simulink model "test"  (R2021b)
settings: Solver=ode1  StartTime=0.0  StopTime=20.0  FixedStep=0.01  RelTol=1e-3
PreLoadFcn:
  | if exist('tl_preloadfcn','file'), tl_preloadfcn(gcs,'5.2.0.25'); end
  | 
  | sDataDefFile = ''; %Empty -> Data Generated into Model source file
  | %% Signal driver_up
  | driver_up = Simulink.Signal;
  | driver_up.DataType = 'boolean';
  | driver_up.Min = 0;
  | driver_up.Max = 1;
  | driver_up.CoderInfo.StorageClass = 'Custom';
  | driver_up.CoderInfo.CustomStorageClass = 'ExportToFile';
  | driver_up.CoderInfo.CustomAttributes.DefinitionFile = sDataDefFile;
  | %% Parameter auto_up_time
  | auto_up_time            = Simulink.Parameter;
  | auto_up_time.Value      = 100;
  | auto_up_time.DataType   = 'uint8';
  | auto_up_time.Min        = 0;
  | auto_up_time.Max        = 255;
  | auto_up_time.CoderInfo.StorageClass = 'Custom';
  | auto_up_time.CoderInfo.CustomStorageClass = 'ConstVolatile';
  | auto_up_time.CoderInfo.CustomAttributes.DefinitionFile = sDataDefFile;
  | %% Signal driver_down
  | driver_down                 = copy(driver_up);
  | %% Signal passenger_up
  | passenger_up                = copy(driver_up);
  | %% Signal passenger_down
  | passenger_down              = copy(driver_up);
  | move_up                     = copy(driver_up);
  | move_down                   = copy(driver_up);
  | obstacle_detection          = copy(driver_up);
  | driver_validated_neutral    = copy(driver_up);
  | driver_validated_up         = copy(driver_up);
  | driver_validated_down       = copy(driver_up);
  | passenger_validated_neutral = copy(driver_up);
  | passenger_validated_up      = copy(driver_up);
  | passenger_validated_down    = copy(driver_up);
  | endstop_top                 = copy(driver_up);
  | endstop_bottom              = copy(driver_up);
  | prev_move_up                = copy(driver_up);
  | obstacle_position = Simulink.Signal;
  | obstacle_position.DataType = 'fixdt(0,16,0.001,0)';
  | obstacle_position.Min = 0;
  | obstacle_position.Max = 0.45;
  | obstacle_position.CoderInfo.StorageClass        = 'Custom';
  | obstacle_position.CoderInfo.CustomStorageClass  = 'ExportToFile';
  | obstacle_position.CoderInfo.CustomAttributes.DefinitionFile = sDataDefFile;
  | 
  | window_position = copy(obstacle_position);
  | 
  | %% Parameters (Global Const Volatile)
  | position_endstop_top            = Simulink.Parameter;
  | position_endstop_top.Value      = 0.4;
  | position_endstop_top.DataType   = 'fixdt(0,16,0.001,0)';
  | position_endstop_top.Min        = 0.35;
  | position_endstop_top.Max        = 0.45;
  | position_endstop_top.CoderInfo.StorageClass = 'Custom';
  | position_endstop_top.CoderInfo.CustomStorageClass = 'ConstVolatile';
  | position_endstop_top.CoderInfo.CustomAttributes.DefinitionFile = sDataDefFile;
  | auto_down_time = copy(auto_up_time);
  | emergency_down_time = copy(auto_up_time);
  | %% Constant
  | ... (+7 lines)
PostLoadFcn:
  | if exist('tl_postloadfcn','file'), tl_postloadfcn(gcs,'5.2.0.25'); end
InitFcn:
  | if exist('tlds_init','file'), tlds_init(gcs); end
StartFcn:
  | if exist('tlds_start','file'), tlds_start(gcs); end
StopFcn:
  | if exist('tlds_stop','file'), tlds_stop(gcs); end
libraries: tllib x7
(part 2 of 2)

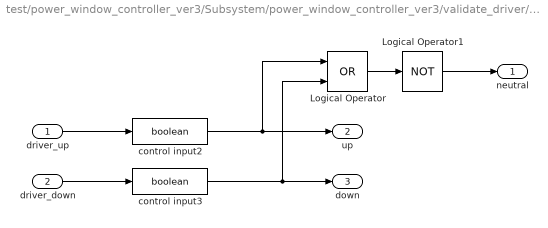
== system test/power_window_controller_ver3/Subsystem/power_window_controller_ver3/validate_driver/driver_switch ==
  driver_up : Inport  RequirementInfo={} %GIDa_88509d42_ace7_45cf_b2c2_89e39ae0ed2c
  driver_down : Inport  RequirementInfo={} %GIDa_beb14dc3_344f_4742_a2d0_fd6ea4a2bf32  Port=2
  Logical Operator : Logic  RequirementInfo={} %GIDa_da5550dd_f94c_4b73_b961_4a47a5203149  Operator=OR  AllPortsSameDT=off  OutDataTypeStr=boolean  mask(TL_LogicalOperator){data={'date',735992.62219250004}}
      settings: CopyFcn=if exist('copy_tlblock','file')==2,copy_tlblock(gcbh);end  DeleteFcn=if exist('delete_tlblock','file')==2,delete_tlblock(gcbh);end  NameChangeFcn=if exist('rename_tlblock','file')==2,rename_tlblock(gcbh);end  OpenFcn=if exist('tl_open_blockdlg','file')==2,tl_open_blockdlg(gcbh);else,open_system(gcbh,'parameter');end
      mask Help: eval(['if exist(''tl_online_help'',''file'') == 2, tl_online_help(''Topic'',''TL_LogicalOperator''),else, web([''jar:file:///'',matlabroot,''/help/toolbox/simulink/help.jar!/slref/' lower(get_param(gcbh,'Blocktype')) '.html''], ''-helpbrowser''),end'])
      mask Display:
      | [x,y] = tlDrawBrandOnBlockIcon(gcbh);
      | plot(x,y);
  Logical Operator1 : Logic  RequirementInfo={} %GIDa_999e8679_8f6d_4720_ab4a_29693e123b6b  Operator=NOT  Inputs=1  AllPortsSameDT=off  OutDataTypeStr=boolean  mask(TL_LogicalOperator){data={'date',735992.62266063655}}
      settings: CopyFcn=if exist('copy_tlblock','file')==2,copy_tlblock(gcbh);end  DeleteFcn=if exist('delete_tlblock','file')==2,delete_tlblock(gcbh);end  NameChangeFcn=if exist('rename_tlblock','file')==2,rename_tlblock(gcbh);end  OpenFcn=if exist('tl_open_blockdlg','file')==2,tl_open_blockdlg(gcbh);else,open_system(gcbh,'parameter');end
      mask Help: eval(['if exist(''tl_online_help'',''file'') == 2, tl_online_help(''Topic'',''TL_LogicalOperator''),else, web([''jar:file:///'',matlabroot,''/help/toolbox/simulink/help.jar!/slref/' lower(get_param(gcbh,'Blocktype')) '.html''], ''-helpbrowser''),end'])
      mask Display:
      | [x,y] = tlDrawBrandOnBlockIcon(gcbh);
      | plot(x,y);
  control input2 : DataTypeConversion  RequirementInfo={} %GIDa_1fd256de_8139_439f_b8bd_b0cd16c1aab9  OutDataTypeStr=boolean  SaturateOnIntegerOverflow=on  RndMeth=Zero  mask(TL_Rescaler){data={'date',730486}}
      settings: CopyFcn=if exist('copy_tlblock','file')==2,copy_tlblock(gcbh);end  DeleteFcn=if exist('delete_tlblock','file')==2,delete_tlblock(gcbh);end  NameChangeFcn=if exist('rename_tlblock','file')==2,rename_tlblock(gcbh);end  OpenFcn=if exist('tl_open_blockdlg','file')==2,tl_open_blockdlg(gcbh);else,open_system(gcbh,'parameter');end
      mask Help: eval(['if exist(''tl_online_help'',''file'') == 2, tl_online_help(''Topic'',''TL_Rescaler''),else, web([''jar:file:///'',matlabroot,''/help/toolbox/simulink/help.jar!/slref/' lower(get_param(gcbh,'Blocktype')) '.html''], ''-helpbrowser''),end'])
      mask Display:
      | [x,y] = tlDrawBrandOnBlockIcon(gcbh);
      | plot(x,y);
  control input3 : DataTypeConversion  RequirementInfo={} %GIDa_36784b95_c4a4_49da_bf15_3958bcd12f2f  OutDataTypeStr=boolean  SaturateOnIntegerOverflow=on  RndMeth=Zero  mask(TL_Rescaler){data={'date',730486}}
      settings: CopyFcn=if exist('copy_tlblock','file')==2,copy_tlblock(gcbh);end  DeleteFcn=if exist('delete_tlblock','file')==2,delete_tlblock(gcbh);end  NameChangeFcn=if exist('rename_tlblock','file')==2,rename_tlblock(gcbh);end  OpenFcn=if exist('tl_open_blockdlg','file')==2,tl_open_blockdlg(gcbh);else,open_system(gcbh,'parameter');end
      mask Help: eval(['if exist(''tl_online_help'',''file'') == 2, tl_online_help(''Topic'',''TL_Rescaler''),else, web([''jar:file:///'',matlabroot,''/help/toolbox/simulink/help.jar!/slref/' lower(get_param(gcbh,'Blocktype')) '.html''], ''-helpbrowser''),end'])
      mask Display:
      | [x,y] = tlDrawBrandOnBlockIcon(gcbh);
      | plot(x,y);
  neutral : Outport  RequirementInfo={} %GIDa_52397442_78d7_49fa_a893_524ae7078fcb  VectorParamsAs1DForOutWhenUnconnected=off
  up : Outport  RequirementInfo={} %GIDa_11ca0414_1b98_43c5_8236_d6cb17915be3  Port=2  VectorParamsAs1DForOutWhenUnconnected=off
  down : Outport  RequirementInfo={} %GIDa_c006668c_2a8f_411c_a55d_2fcf10c84114  Port=3  VectorParamsAs1DForOutWhenUnconnected=off
  wires:
  Logical Operator1/1 -> neutral/1
  Logical Operator/1 -> Logical Operator1/1
  control input3/1 -> Logical Operator/2, down/1
  control input2/1 -> Logical Operator/1, up/1
  driver_down/1 -> control input3/1
  driver_up/1 -> control input2/1

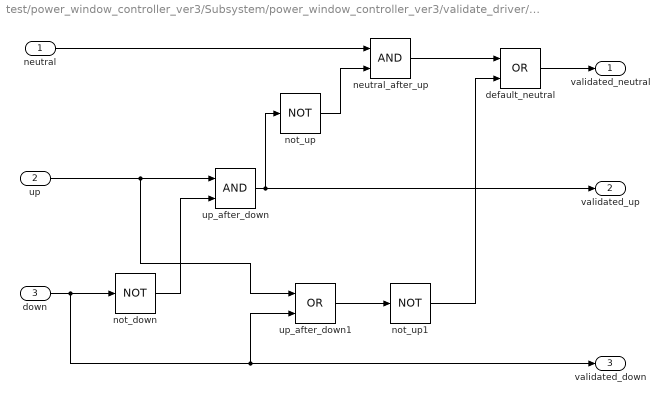
== system test/power_window_controller_ver3/Subsystem/power_window_controller_ver3/validate_driver/mutually_exclusive ==
  neutral : Inport  RequirementInfo={} %GIDa_383a4fa9_ecde_419e_b29b_a733e5593bc2
  up : Inport  RequirementInfo={} %GIDa_3190656b_05c4_4e8f_afb6_15ac29bcab83  Port=2
  down : Inport  RequirementInfo={} %GIDa_9b767e83_1086_482d_996f_d13516317d5e  Port=3
  default_neutral : Logic  RequirementInfo={} %GIDa_d3e9b556_6fe4_4d4f_868e_156175e008c8  Operator=OR  AllPortsSameDT=off  OutDataTypeStr=boolean  mask(TL_LogicalOperator){data={'date',735992.62933622685}}
      settings: CopyFcn=if exist('copy_tlblock','file')==2,copy_tlblock(gcbh);end  DeleteFcn=if exist('delete_tlblock','file')==2,delete_tlblock(gcbh);end  NameChangeFcn=if exist('rename_tlblock','file')==2,rename_tlblock(gcbh);end  OpenFcn=if exist('tl_open_blockdlg','file')==2,tl_open_blockdlg(gcbh);else,open_system(gcbh,'parameter');end
      mask Help: eval(['if exist(''tl_online_help'',''file'') == 2, tl_online_help(''Topic'',''TL_LogicalOperator''),else, web([''jar:file:///'',matlabroot,''/help/toolbox/simulink/help.jar!/slref/' lower(get_param(gcbh,'Blocktype')) '.html''], ''-helpbrowser''),end'])
      mask Display:
      | [x,y] = tlDrawBrandOnBlockIcon(gcbh);
      | plot(x,y);
  neutral_after_up : Logic  RequirementInfo={} %GIDa_2a0ebed4_26f4_4b16_ab66_395a1ddbb03e  AllPortsSameDT=off  OutDataTypeStr=boolean  mask(TL_LogicalOperator){data={'date',730486}}
      settings: CopyFcn=if exist('copy_tlblock','file')==2,copy_tlblock(gcbh);end  DeleteFcn=if exist('delete_tlblock','file')==2,delete_tlblock(gcbh);end  NameChangeFcn=if exist('rename_tlblock','file')==2,rename_tlblock(gcbh);end  OpenFcn=if exist('tl_open_blockdlg','file')==2,tl_open_blockdlg(gcbh);else,open_system(gcbh,'parameter');end
      mask Help: eval(['if exist(''tl_online_help'',''file'') == 2, tl_online_help(''Topic'',''TL_LogicalOperator''),else, web([''jar:file:///'',matlabroot,''/help/toolbox/simulink/help.jar!/slref/' lower(get_param(gcbh,'Blocktype')) '.html''], ''-helpbrowser''),end'])
      mask Display:
      | [x,y] = tlDrawBrandOnBlockIcon(gcbh);
      | plot(x,y);
  not_down : Logic  RequirementInfo={} %GIDa_717def5e_3a6b_41f3_97d3_f7d9ab03bba7  Operator=NOT  Inputs=1  AllPortsSameDT=off  OutDataTypeStr=boolean  mask(TL_LogicalOperator){data={'date',735992.6300086343}}
      settings: CopyFcn=if exist('copy_tlblock','file')==2,copy_tlblock(gcbh);end  DeleteFcn=if exist('delete_tlblock','file')==2,delete_tlblock(gcbh);end  NameChangeFcn=if exist('rename_tlblock','file')==2,rename_tlblock(gcbh);end  OpenFcn=if exist('tl_open_blockdlg','file')==2,tl_open_blockdlg(gcbh);else,open_system(gcbh,'parameter');end
      mask Help: eval(['if exist(''tl_online_help'',''file'') == 2, tl_online_help(''Topic'',''TL_LogicalOperator''),else, web([''jar:file:///'',matlabroot,''/help/toolbox/simulink/help.jar!/slref/' lower(get_param(gcbh,'Blocktype')) '.html''], ''-helpbrowser''),end'])
      mask Display:
      | [x,y] = tlDrawBrandOnBlockIcon(gcbh);
      | plot(x,y);
  not_up : Logic  RequirementInfo={} %GIDa_639c22ba_cf00_4eaa_845a_300072015885  Operator=NOT  Inputs=1  AllPortsSameDT=off  OutDataTypeStr=boolean  mask(TL_LogicalOperator){data={'date',735992.62898631941}}
      settings: CopyFcn=if exist('copy_tlblock','file')==2,copy_tlblock(gcbh);end  DeleteFcn=if exist('delete_tlblock','file')==2,delete_tlblock(gcbh);end  NameChangeFcn=if exist('rename_tlblock','file')==2,rename_tlblock(gcbh);end  OpenFcn=if exist('tl_open_blockdlg','file')==2,tl_open_blockdlg(gcbh);else,open_system(gcbh,'parameter');end
      mask Help: eval(['if exist(''tl_online_help'',''file'') == 2, tl_online_help(''Topic'',''TL_LogicalOperator''),else, web([''jar:file:///'',matlabroot,''/help/toolbox/simulink/help.jar!/slref/' lower(get_param(gcbh,'Blocktype')) '.html''], ''-helpbrowser''),end'])
      mask Display:
      | [x,y] = tlDrawBrandOnBlockIcon(gcbh);
      | plot(x,y);
  not_up1 : Logic  RequirementInfo={} %GIDa_b9044636_34db_4ac8_92ea_fff124b8872b  Operator=NOT  Inputs=1  AllPortsSameDT=off  OutDataTypeStr=boolean  mask(TL_LogicalOperator){data={'date',735992.62922876154}}
      settings: CopyFcn=if exist('copy_tlblock','file')==2,copy_tlblock(gcbh);end  DeleteFcn=if exist('delete_tlblock','file')==2,delete_tlblock(gcbh);end  NameChangeFcn=if exist('rename_tlblock','file')==2,rename_tlblock(gcbh);end  OpenFcn=if exist('tl_open_blockdlg','file')==2,tl_open_blockdlg(gcbh);else,open_system(gcbh,'parameter');end
      mask Help: eval(['if exist(''tl_online_help'',''file'') == 2, tl_online_help(''Topic'',''TL_LogicalOperator''),else, web([''jar:file:///'',matlabroot,''/help/toolbox/simulink/help.jar!/slref/' lower(get_param(gcbh,'Blocktype')) '.html''], ''-helpbrowser''),end'])
      mask Display:
      | [x,y] = tlDrawBrandOnBlockIcon(gcbh);
      | plot(x,y);
  up_after_down : Logic  RequirementInfo={} %GIDa_dfbd8cd7_4a86_47e2_b815_023cc02ff9b3  AllPortsSameDT=off  OutDataTypeStr=boolean  mask(TL_LogicalOperator){data={'date',730486}}
      settings: CopyFcn=if exist('copy_tlblock','file')==2,copy_tlblock(gcbh);end  DeleteFcn=if exist('delete_tlblock','file')==2,delete_tlblock(gcbh);end  NameChangeFcn=if exist('rename_tlblock','file')==2,rename_tlblock(gcbh);end  OpenFcn=if exist('tl_open_blockdlg','file')==2,tl_open_blockdlg(gcbh);else,open_system(gcbh,'parameter');end
      mask Help: eval(['if exist(''tl_online_help'',''file'') == 2, tl_online_help(''Topic'',''TL_LogicalOperator''),else, web([''jar:file:///'',matlabroot,''/help/toolbox/simulink/help.jar!/slref/' lower(get_param(gcbh,'Blocktype')) '.html''], ''-helpbrowser''),end'])
      mask Display:
      | [x,y] = tlDrawBrandOnBlockIcon(gcbh);
      | plot(x,y);
  up_after_down1 : Logic  RequirementInfo={} %GIDa_d95a3b1c_b63e_4679_81b0_52373f842e5a  Operator=OR  AllPortsSameDT=off  OutDataTypeStr=boolean  mask(TL_LogicalOperator){data={'date',735992.62915869209}}
      settings: CopyFcn=if exist('copy_tlblock','file')==2,copy_tlblock(gcbh);end  DeleteFcn=if exist('delete_tlblock','file')==2,delete_tlblock(gcbh);end  NameChangeFcn=if exist('rename_tlblock','file')==2,rename_tlblock(gcbh);end  OpenFcn=if exist('tl_open_blockdlg','file')==2,tl_open_blockdlg(gcbh);else,open_system(gcbh,'parameter');end
      mask Help: eval(['if exist(''tl_online_help'',''file'') == 2, tl_online_help(''Topic'',''TL_LogicalOperator''),else, web([''jar:file:///'',matlabroot,''/help/toolbox/simulink/help.jar!/slref/' lower(get_param(gcbh,'Blocktype')) '.html''], ''-helpbrowser''),end'])
      mask Display:
      | [x,y] = tlDrawBrandOnBlockIcon(gcbh);
      | plot(x,y);
  validated_neutral : Outport  RequirementInfo={} %GIDa_3c0727ef_8ebe_4a26_9872_7ecff81cc607  VectorParamsAs1DForOutWhenUnconnected=off
  validated_up : Outport  RequirementInfo={} %GIDa_19324167_0f79_4534_b0cb_f13c4416581a  Port=2  VectorParamsAs1DForOutWhenUnconnected=off
  validated_down : Outport  RequirementInfo={} %GIDa_0162b81e_3c7a_4e42_9ca4_e1cfc5546455  Port=3  VectorParamsAs1DForOutWhenUnconnected=off
  wires:
  default_neutral/1 -> validated_neutral/1
  neutral_after_up/1 -> default_neutral/1
  not_up1/1 -> default_neutral/2
  up_after_down1/1 -> not_up1/1
  not_down/1 -> up_after_down/2
  down/1 -> up_after_down1/2, validated_down/1, not_down/1
  up/1 -> up_after_down1/1, up_after_down/1
  up_after_down/1 -> not_up/1, validated_up/1
  not_up/1 -> neutral_after_up/2
  neutral/1 -> neutral_after_up/1

== system test/power_window_controller_ver3/Subsystem/power_window_controller_ver3/validate_passenger/check_down ==
  action : Inport  RequirementInfo={} %GIDa_da076438_353a_470e_9b80_f82c98211ee1
  endstop : Inport  RequirementInfo={} %GIDa_ce714160_616b_4c6d_8540_ba9727262a40  Port=2
  allow_action : Logic  RequirementInfo={} %GIDa_fe6c6090_dc3d_4b4b_8e5b_0840ba53ae61  AllPortsSameDT=off  OutDataTypeStr=boolean  mask(TL_LogicalOperator){data={'date',730486}}
      settings: CopyFcn=if exist('copy_tlblock','file')==2,copy_tlblock(gcbh);end  DeleteFcn=if exist('delete_tlblock','file')==2,delete_tlblock(gcbh);end  NameChangeFcn=if exist('rename_tlblock','file')==2,rename_tlblock(gcbh);end  OpenFcn=if exist('tl_open_blockdlg','file')==2,tl_open_blockdlg(gcbh);else,open_system(gcbh,'parameter');end
      mask Help: eval(['if exist(''tl_online_help'',''file'') == 2, tl_online_help(''Topic'',''TL_LogicalOperator''),else, web([''jar:file:///'',matlabroot,''/help/toolbox/simulink/help.jar!/slref/' lower(get_param(gcbh,'Blocktype')) '.html''], ''-helpbrowser''),end'])
      mask Display:
      | [x,y] = tlDrawBrandOnBlockIcon(gcbh);
      | plot(x,y);
  not : Logic  RequirementInfo={} %GIDa_533718db_3046_4631_b21c_e5e46c0b500e  Operator=NOT  Inputs=1  AllPortsSameDT=off  OutDataTypeStr=boolean  mask(TL_LogicalOperator){data={'date',735992.64851342596}}
      settings: CopyFcn=if exist('copy_tlblock','file')==2,copy_tlblock(gcbh);end  DeleteFcn=if exist('delete_tlblock','file')==2,delete_tlblock(gcbh);end  NameChangeFcn=if exist('rename_tlblock','file')==2,rename_tlblock(gcbh);end  OpenFcn=if exist('tl_open_blockdlg','file')==2,tl_open_blockdlg(gcbh);else,open_system(gcbh,'parameter');end
      mask Help: eval(['if exist(''tl_online_help'',''file'') == 2, tl_online_help(''Topic'',''TL_LogicalOperator''),else, web([''jar:file:///'',matlabroot,''/help/toolbox/simulink/help.jar!/slref/' lower(get_param(gcbh,'Blocktype')) '.html''], ''-helpbrowser''),end'])
      mask Display:
      | [x,y] = tlDrawBrandOnBlockIcon(gcbh);
      | plot(x,y);
  checked_action : Outport  RequirementInfo={} %GIDa_6c5fa107_9f31_4e7d_b1d4_63d44d132e8c  VectorParamsAs1DForOutWhenUnconnected=off
  wires:
  action/1 -> allow_action/1
  not/1 -> allow_action/2
  allow_action/1 -> checked_action/1  "checked_action"
  endstop/1 -> not/1

== system test/power_window_controller_ver3/Subsystem/power_window_controller_ver3/validate_passenger/check_up ==
  action : Inport  RequirementInfo={} %GIDa_f59cf256_ba50_4778_a7ea_a9838d29ca65
  endstop : Inport  RequirementInfo={} %GIDa_faea268d_9968_4a7f_be13_1dc8cf9d81cc  Port=2
  allow_action : Logic  RequirementInfo={} %GIDa_bdf451d4_0a10_4233_9fa7_d183d3ea2ff8  AllPortsSameDT=off  OutDataTypeStr=boolean  mask(TL_LogicalOperator){data={'date',730486}}
      settings: CopyFcn=if exist('copy_tlblock','file')==2,copy_tlblock(gcbh);end  DeleteFcn=if exist('delete_tlblock','file')==2,delete_tlblock(gcbh);end  NameChangeFcn=if exist('rename_tlblock','file')==2,rename_tlblock(gcbh);end  OpenFcn=if exist('tl_open_blockdlg','file')==2,tl_open_blockdlg(gcbh);else,open_system(gcbh,'parameter');end
      mask Help: eval(['if exist(''tl_online_help'',''file'') == 2, tl_online_help(''Topic'',''TL_LogicalOperator''),else, web([''jar:file:///'',matlabroot,''/help/toolbox/simulink/help.jar!/slref/' lower(get_param(gcbh,'Blocktype')) '.html''], ''-helpbrowser''),end'])
      mask Display:
      | [x,y] = tlDrawBrandOnBlockIcon(gcbh);
      | plot(x,y);
  not : Logic  RequirementInfo={} %GIDa_f616a659_3f71_45f7_a114_87f81250fdbe  Operator=NOT  Inputs=1  AllPortsSameDT=off  OutDataTypeStr=boolean  mask(TL_LogicalOperator){data={'date',735992.62481011578}}
      settings: CopyFcn=if exist('copy_tlblock','file')==2,copy_tlblock(gcbh);end  DeleteFcn=if exist('delete_tlblock','file')==2,delete_tlblock(gcbh);end  NameChangeFcn=if exist('rename_tlblock','file')==2,rename_tlblock(gcbh);end  OpenFcn=if exist('tl_open_blockdlg','file')==2,tl_open_blockdlg(gcbh);else,open_system(gcbh,'parameter');end
      mask Help: eval(['if exist(''tl_online_help'',''file'') == 2, tl_online_help(''Topic'',''TL_LogicalOperator''),else, web([''jar:file:///'',matlabroot,''/help/toolbox/simulink/help.jar!/slref/' lower(get_param(gcbh,'Blocktype')) '.html''], ''-helpbrowser''),end'])
      mask Display:
      | [x,y] = tlDrawBrandOnBlockIcon(gcbh);
      | plot(x,y);
  checked_action : Outport  RequirementInfo={} %GIDa_b43b2120_3294_45de_be03_5247a9810093  VectorParamsAs1DForOutWhenUnconnected=off
  wires:
  not/1 -> allow_action/2
  endstop/1 -> not/1
  action/1 -> allow_action/1
  allow_action/1 -> checked_action/1  "checked_action"

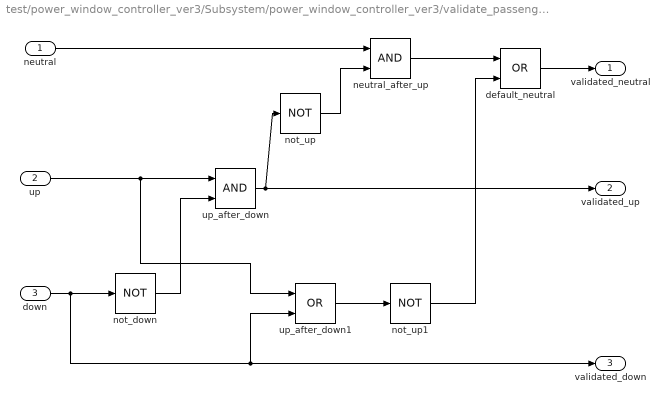
== system test/power_window_controller_ver3/Subsystem/power_window_controller_ver3/validate_passenger/mutually_exclusive ==
  neutral : Inport  RequirementInfo={} %GIDa_424a211a_6df5_4483_bfdf_defbb12d93f1
  up : Inport  RequirementInfo={} %GIDa_33e8d64b_ac9c_4095_99e6_971b64359682  Port=2
  down : Inport  RequirementInfo={} %GIDa_7e89cca4_8fef_4b9e_9225_2b9b9d3c5aac  Port=3
  default_neutral : Logic  RequirementInfo={} %GIDa_8acc70e5_66ec_4e5d_9241_19446d74547b  Operator=OR  AllPortsSameDT=off  OutDataTypeStr=boolean  mask(TL_LogicalOperator){data={'date',735992.62933622685}}
      settings: CopyFcn=if exist('copy_tlblock','file')==2,copy_tlblock(gcbh);end  DeleteFcn=if exist('delete_tlblock','file')==2,delete_tlblock(gcbh);end  NameChangeFcn=if exist('rename_tlblock','file')==2,rename_tlblock(gcbh);end  OpenFcn=if exist('tl_open_blockdlg','file')==2,tl_open_blockdlg(gcbh);else,open_system(gcbh,'parameter');end
      mask Help: eval(['if exist(''tl_online_help'',''file'') == 2, tl_online_help(''Topic'',''TL_LogicalOperator''),else, web([''jar:file:///'',matlabroot,''/help/toolbox/simulink/help.jar!/slref/' lower(get_param(gcbh,'Blocktype')) '.html''], ''-helpbrowser''),end'])
      mask Display:
      | [x,y] = tlDrawBrandOnBlockIcon(gcbh);
      | plot(x,y);
  neutral_after_up : Logic  RequirementInfo={} %GIDa_69f8b653_9e13_44eb_8f1b_d1f3ae125580  AllPortsSameDT=off  OutDataTypeStr=boolean  mask(TL_LogicalOperator){data={'date',730486}}
      settings: CopyFcn=if exist('copy_tlblock','file')==2,copy_tlblock(gcbh);end  DeleteFcn=if exist('delete_tlblock','file')==2,delete_tlblock(gcbh);end  NameChangeFcn=if exist('rename_tlblock','file')==2,rename_tlblock(gcbh);end  OpenFcn=if exist('tl_open_blockdlg','file')==2,tl_open_blockdlg(gcbh);else,open_system(gcbh,'parameter');end
      mask Help: eval(['if exist(''tl_online_help'',''file'') == 2, tl_online_help(''Topic'',''TL_LogicalOperator''),else, web([''jar:file:///'',matlabroot,''/help/toolbox/simulink/help.jar!/slref/' lower(get_param(gcbh,'Blocktype')) '.html''], ''-helpbrowser''),end'])
      mask Display:
      | [x,y] = tlDrawBrandOnBlockIcon(gcbh);
      | plot(x,y);
  not_down : Logic  RequirementInfo={} %GIDa_d1d7b344_57a6_42b5_b93a_d340b43b1746  Operator=NOT  Inputs=1  AllPortsSameDT=off  OutDataTypeStr=boolean  mask(TL_LogicalOperator){data={'date',735992.6300086343}}
      settings: CopyFcn=if exist('copy_tlblock','file')==2,copy_tlblock(gcbh);end  DeleteFcn=if exist('delete_tlblock','file')==2,delete_tlblock(gcbh);end  NameChangeFcn=if exist('rename_tlblock','file')==2,rename_tlblock(gcbh);end  OpenFcn=if exist('tl_open_blockdlg','file')==2,tl_open_blockdlg(gcbh);else,open_system(gcbh,'parameter');end
      mask Help: eval(['if exist(''tl_online_help'',''file'') == 2, tl_online_help(''Topic'',''TL_LogicalOperator''),else, web([''jar:file:///'',matlabroot,''/help/toolbox/simulink/help.jar!/slref/' lower(get_param(gcbh,'Blocktype')) '.html''], ''-helpbrowser''),end'])
      mask Display:
      | [x,y] = tlDrawBrandOnBlockIcon(gcbh);
      | plot(x,y);
  not_up : Logic  RequirementInfo={} %GIDa_9c15ceaf_c029_4c35_b6f7_26fc8d50536e  Operator=NOT  Inputs=1  AllPortsSameDT=off  OutDataTypeStr=boolean  mask(TL_LogicalOperator){data={'date',735992.62898631941}}
      settings: CopyFcn=if exist('copy_tlblock','file')==2,copy_tlblock(gcbh);end  DeleteFcn=if exist('delete_tlblock','file')==2,delete_tlblock(gcbh);end  NameChangeFcn=if exist('rename_tlblock','file')==2,rename_tlblock(gcbh);end  OpenFcn=if exist('tl_open_blockdlg','file')==2,tl_open_blockdlg(gcbh);else,open_system(gcbh,'parameter');end
      mask Help: eval(['if exist(''tl_online_help'',''file'') == 2, tl_online_help(''Topic'',''TL_LogicalOperator''),else, web([''jar:file:///'',matlabroot,''/help/toolbox/simulink/help.jar!/slref/' lower(get_param(gcbh,'Blocktype')) '.html''], ''-helpbrowser''),end'])
      mask Display:
      | [x,y] = tlDrawBrandOnBlockIcon(gcbh);
      | plot(x,y);
  not_up1 : Logic  RequirementInfo={} %GIDa_ce662c6d_fc19_42f3_9dbb_1a05731d89ca  Operator=NOT  Inputs=1  AllPortsSameDT=off  OutDataTypeStr=boolean  mask(TL_LogicalOperator){data={'date',735992.62922876154}}
      settings: CopyFcn=if exist('copy_tlblock','file')==2,copy_tlblock(gcbh);end  DeleteFcn=if exist('delete_tlblock','file')==2,delete_tlblock(gcbh);end  NameChangeFcn=if exist('rename_tlblock','file')==2,rename_tlblock(gcbh);end  OpenFcn=if exist('tl_open_blockdlg','file')==2,tl_open_blockdlg(gcbh);else,open_system(gcbh,'parameter');end
      mask Help: eval(['if exist(''tl_online_help'',''file'') == 2, tl_online_help(''Topic'',''TL_LogicalOperator''),else, web([''jar:file:///'',matlabroot,''/help/toolbox/simulink/help.jar!/slref/' lower(get_param(gcbh,'Blocktype')) '.html''], ''-helpbrowser''),end'])
      mask Display:
      | [x,y] = tlDrawBrandOnBlockIcon(gcbh);
      | plot(x,y);
  up_after_down : Logic  RequirementInfo={} %GIDa_16be3082_a051_4113_8ebd_5084a1f9543d  AllPortsSameDT=off  OutDataTypeStr=boolean  mask(TL_LogicalOperator){data={'date',730486}}
      settings: CopyFcn=if exist('copy_tlblock','file')==2,copy_tlblock(gcbh);end  DeleteFcn=if exist('delete_tlblock','file')==2,delete_tlblock(gcbh);end  NameChangeFcn=if exist('rename_tlblock','file')==2,rename_tlblock(gcbh);end  OpenFcn=if exist('tl_open_blockdlg','file')==2,tl_open_blockdlg(gcbh);else,open_system(gcbh,'parameter');end
      mask Help: eval(['if exist(''tl_online_help'',''file'') == 2, tl_online_help(''Topic'',''TL_LogicalOperator''),else, web([''jar:file:///'',matlabroot,''/help/toolbox/simulink/help.jar!/slref/' lower(get_param(gcbh,'Blocktype')) '.html''], ''-helpbrowser''),end'])
      mask Display:
      | [x,y] = tlDrawBrandOnBlockIcon(gcbh);
      | plot(x,y);
  up_after_down1 : Logic  RequirementInfo={} %GIDa_db007b8f_3830_466d_a6f6_c59c0124e08e  Operator=OR  AllPortsSameDT=off  OutDataTypeStr=boolean  mask(TL_LogicalOperator){data={'date',735992.62915869209}}
      settings: CopyFcn=if exist('copy_tlblock','file')==2,copy_tlblock(gcbh);end  DeleteFcn=if exist('delete_tlblock','file')==2,delete_tlblock(gcbh);end  NameChangeFcn=if exist('rename_tlblock','file')==2,rename_tlblock(gcbh);end  OpenFcn=if exist('tl_open_blockdlg','file')==2,tl_open_blockdlg(gcbh);else,open_system(gcbh,'parameter');end
      mask Help: eval(['if exist(''tl_online_help'',''file'') == 2, tl_online_help(''Topic'',''TL_LogicalOperator''),else, web([''jar:file:///'',matlabroot,''/help/toolbox/simulink/help.jar!/slref/' lower(get_param(gcbh,'Blocktype')) '.html''], ''-helpbrowser''),end'])
      mask Display:
      | [x,y] = tlDrawBrandOnBlockIcon(gcbh);
      | plot(x,y);
  validated_neutral : Outport  RequirementInfo={} %GIDa_c34df9a8_faa3_4845_b234_d783233c3629  VectorParamsAs1DForOutWhenUnconnected=off
  validated_up : Outport  RequirementInfo={} %GIDa_467ffbc7_d904_4b58_ba02_3479a23c2a13  Port=2  VectorParamsAs1DForOutWhenUnconnected=off
  validated_down : Outport  RequirementInfo={} %GIDa_5d315801_0d6f_41f7_9a4a_92c389cb8d22  Port=3  VectorParamsAs1DForOutWhenUnconnected=off
  wires:
  default_neutral/1 -> validated_neutral/1
  neutral_after_up/1 -> default_neutral/1
  not_up1/1 -> default_neutral/2
  up_after_down1/1 -> not_up1/1
  not_down/1 -> up_after_down/2
  down/1 -> up_after_down1/2, validated_down/1, not_down/1
  up/1 -> up_after_down1/1, up_after_down/1
  up_after_down/1 -> not_up/1, validated_up/1
  not_up/1 -> neutral_after_up/2
  neutral/1 -> neutral_after_up/1

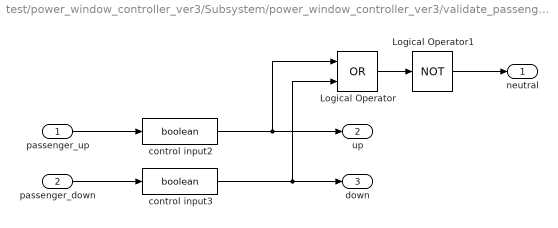
== system test/power_window_controller_ver3/Subsystem/power_window_controller_ver3/validate_passenger/passenger_switch ==
  passenger_up : Inport  RequirementInfo={} %GIDa_5194764c_b274_4fd9_bc4b_626bd3c498dd
  passenger_down : Inport  RequirementInfo={} %GIDa_31df0a05_cb75_4a47_ae8a_08b0e9241ed4  Port=2
  Logical Operator : Logic  RequirementInfo={} %GIDa_68e262f7_493a_4897_9b58_059992e92e41  Operator=OR  AllPortsSameDT=off  OutDataTypeStr=boolean  mask(TL_LogicalOperator){data={'date',735992.62219250004}}
      settings: CopyFcn=if exist('copy_tlblock','file')==2,copy_tlblock(gcbh);end  DeleteFcn=if exist('delete_tlblock','file')==2,delete_tlblock(gcbh);end  NameChangeFcn=if exist('rename_tlblock','file')==2,rename_tlblock(gcbh);end  OpenFcn=if exist('tl_open_blockdlg','file')==2,tl_open_blockdlg(gcbh);else,open_system(gcbh,'parameter');end
      mask Help: eval(['if exist(''tl_online_help'',''file'') == 2, tl_online_help(''Topic'',''TL_LogicalOperator''),else, web([''jar:file:///'',matlabroot,''/help/toolbox/simulink/help.jar!/slref/' lower(get_param(gcbh,'Blocktype')) '.html''], ''-helpbrowser''),end'])
      mask Display:
      | [x,y] = tlDrawBrandOnBlockIcon(gcbh);
      | plot(x,y);
  Logical Operator1 : Logic  RequirementInfo={} %GIDa_b09a42c5_557d_4371_b994_f058452ca5d4  Operator=NOT  Inputs=1  AllPortsSameDT=off  OutDataTypeStr=boolean  mask(TL_LogicalOperator){data={'date',735992.62266063655}}
      settings: CopyFcn=if exist('copy_tlblock','file')==2,copy_tlblock(gcbh);end  DeleteFcn=if exist('delete_tlblock','file')==2,delete_tlblock(gcbh);end  NameChangeFcn=if exist('rename_tlblock','file')==2,rename_tlblock(gcbh);end  OpenFcn=if exist('tl_open_blockdlg','file')==2,tl_open_blockdlg(gcbh);else,open_system(gcbh,'parameter');end
      mask Help: eval(['if exist(''tl_online_help'',''file'') == 2, tl_online_help(''Topic'',''TL_LogicalOperator''),else, web([''jar:file:///'',matlabroot,''/help/toolbox/simulink/help.jar!/slref/' lower(get_param(gcbh,'Blocktype')) '.html''], ''-helpbrowser''),end'])
      mask Display:
      | [x,y] = tlDrawBrandOnBlockIcon(gcbh);
      | plot(x,y);
  control input2 : DataTypeConversion  RequirementInfo={} %GIDa_010a16a9_4eb9_482b_9082_d2aac13b41b2  OutDataTypeStr=boolean  SaturateOnIntegerOverflow=on  RndMeth=Zero  mask(TL_Rescaler){data={'date',730486}}
      settings: CopyFcn=if exist('copy_tlblock','file')==2,copy_tlblock(gcbh);end  DeleteFcn=if exist('delete_tlblock','file')==2,delete_tlblock(gcbh);end  NameChangeFcn=if exist('rename_tlblock','file')==2,rename_tlblock(gcbh);end  OpenFcn=if exist('tl_open_blockdlg','file')==2,tl_open_blockdlg(gcbh);else,open_system(gcbh,'parameter');end
      mask Help: eval(['if exist(''tl_online_help'',''file'') == 2, tl_online_help(''Topic'',''TL_Rescaler''),else, web([''jar:file:///'',matlabroot,''/help/toolbox/simulink/help.jar!/slref/' lower(get_param(gcbh,'Blocktype')) '.html''], ''-helpbrowser''),end'])
      mask Display:
      | [x,y] = tlDrawBrandOnBlockIcon(gcbh);
      | plot(x,y);
  control input3 : DataTypeConversion  RequirementInfo={} %GIDa_1854ba8c_a1f2_4ce0_a9d9_9bb09b7a8ce9  OutDataTypeStr=boolean  SaturateOnIntegerOverflow=on  RndMeth=Zero  mask(TL_Rescaler){data={'date',730486}}
      settings: CopyFcn=if exist('copy_tlblock','file')==2,copy_tlblock(gcbh);end  DeleteFcn=if exist('delete_tlblock','file')==2,delete_tlblock(gcbh);end  NameChangeFcn=if exist('rename_tlblock','file')==2,rename_tlblock(gcbh);end  OpenFcn=if exist('tl_open_blockdlg','file')==2,tl_open_blockdlg(gcbh);else,open_system(gcbh,'parameter');end
      mask Help: eval(['if exist(''tl_online_help'',''file'') == 2, tl_online_help(''Topic'',''TL_Rescaler''),else, web([''jar:file:///'',matlabroot,''/help/toolbox/simulink/help.jar!/slref/' lower(get_param(gcbh,'Blocktype')) '.html''], ''-helpbrowser''),end'])
      mask Display:
      | [x,y] = tlDrawBrandOnBlockIcon(gcbh);
      | plot(x,y);
  neutral : Outport  RequirementInfo={} %GIDa_595a0280_f1a8_42d5_b11f_31fbaec81abf  VectorParamsAs1DForOutWhenUnconnected=off
  up : Outport  RequirementInfo={} %GIDa_488607ed_1f67_4afb_bb62_2e440ef8d475  Port=2  VectorParamsAs1DForOutWhenUnconnected=off
  down : Outport  RequirementInfo={} %GIDa_63154fdf_e9ae_4f4a_bf1e_53d87031dba5  Port=3  VectorParamsAs1DForOutWhenUnconnected=off
  wires:
  Logical Operator1/1 -> neutral/1
  Logical Operator/1 -> Logical Operator1/1
  control input3/1 -> Logical Operator/2, down/1
  control input2/1 -> Logical Operator/1, up/1
  passenger_down/1 -> control input3/1
  passenger_up/1 -> control input2/1

== stateflow chart test/power_window_controller_ver3/Subsystem/power_window_controller_ver3/control ==
  state safe
    state driverNeutral
      entry:
      moveUp = 0;
      moveDown = 0;
      state passengerneutral
        entry:
        moveUp = 0;
        moveDown = 0;
      state passengerDown
        entry: moveDown = 1;
        exit:   moveDown = 0;
        state iniPassengerDown
        state passengerDown
        state autoPassengerDown
        iniPassengerDown -> (junction 14) : after(auto_down_time,tick)
        (junction 14) -> safe.driverNeutral.passengerDown.passengerDown [order 2]
        (junction 14) -> autoPassengerDown [order 1] : [passenger_neutral]
      state passengerUp
        entry: moveUp = 1;
        exit: moveUp = 0;
        state iniPassengerUp
        state PassengerUp
        state autoPassengerUp
        iniPassengerUp -> (junction 29) : after(auto_up_time,tick)
        (junction 29) -> PassengerUp [order 2]
        (junction 29) -> autoPassengerUp [order 1] : [passenger_neutral]
      (default) -> passengerneutral
      passengerneutral -> iniPassengerUp [order 1] : [passenger_up]
      passengerneutral -> iniPassengerDown [order 2] : [passenger_down]
      safe.driverNeutral.passengerDown.passengerDown -> passengerneutral : [passenger_neutral]
      PassengerUp -> passengerneutral : [passenger_neutral]
      safe.driverNeutral.passengerDown -> passengerneutral [order 1] : [endstop_bottom]
      passengerUp -> passengerneutral [order 2] : [endstop_top]
      safe.driverNeutral.passengerDown -> PassengerUp [order 2] : [passenger_up]
      passengerUp -> safe.driverNeutral.passengerDown.passengerDown [order 1] : [passenger_down]
    state driverUp
      entry: moveUp = 1;
      exit: moveUp = 0;
      state iniDriverUp
      state DriverUp
      state autoDriverUp
      iniDriverUp -> (junction 55) : after(auto_up_time,tick)
      (junction 55) -> DriverUp [order 2]
      (junction 55) -> autoDriverUp [order 1] : [driver_neutral]
    state driverDown
      entry: moveDown = 1;
      exit: moveDown = 0;
      state iniDriverDown
      state DriverDown
      state autoDriverDown
      iniDriverDown -> (junction 44) : after(auto_down_time,tick)
      (junction 44) -> DriverDown [order 2]
      (junction 44) -> autoDriverDown [order 1] : [driver_neutral]
    (default) -> driverNeutral
    driverNeutral -> iniDriverDown [order 3] : [driver_down]
    DriverDown -> driverNeutral : [driver_neutral]
    driverDown -> driverNeutral [order 1] : [endstop_bottom]
    DriverUp -> driverNeutral : [driver_neutral]
    driverUp -> driverNeutral [order 2] : [endstop_top]
    driverNeutral -> iniDriverUp [order 2] : [driver_up]
    driverDown -> DriverUp [order 2] : [driver_up]
    driverUp -> DriverDown [order 1] : [driver_down]
  state emergencyDown
    entry:
    moveUp = 0;
    moveDown = 1;
  emergencyDown -> passengerneutral : [endstop_bottom | after(emergency_down_time,tick)]
  (default) -> safe
  driverNeutral -> emergencyDown [order 1] : [obstacle]
  data: auto_up_time input; auto_down_time input; emergency_down_time input; driver_neutral input; driver_up input; driver_down input; passenger_neutral input; passenger_up input; passenger_down input; obstacle input; endstop_bottom input; endstop_top input; moveDown output double; moveUp output
  data auto_up_time settings: description=$TL$ type=UInt8; date=20170127T121040; $TL$
  data auto_down_time settings: description=$TL$ type=UInt8; date=20170127T121041; $TL$
  data emergency_down_time settings: description=$TL$ type=UInt8; date=20170127T121041; $TL$
  data driver_neutral settings: description=$TL$ type=Bool; $TL$
  data driver_up settings: description=$TL$ type=Bool; $TL$
  data driver_down settings: description=$TL$ type=Bool; $TL$
  data passenger_neutral settings: description=$TL$ type=Bool; $TL$
  data passenger_up settings: description=$TL$ type=Bool; $TL$
  data passenger_down settings: description=$TL$ type=Bool; $TL$
  data obstacle settings: description=$TL$ type=Bool; $TL$
  data endstop_bottom settings: description=$TL$ type=Bool; $TL$
  data endstop_top settings: description=$TL$ type=Bool; $TL$
  data moveDown settings: description=$TL$ type=Bool; date=20170127T121045; $TL$
  data moveUp settings: description=$TL$ type=Bool; date=20170127T121045; $TL$
